simulink model "s_c856m4k_cd"  (R2016b)
(part 21 of 60)

  rx_crc_err_lnk3 : Subsystem  Tag=xps:sw_reg  AncestorBlock=xps_library/software_register  mask(swreg){io_dir=To Processor, io_delay=0, sample_period=1, names=reg, bitwidths=16, bin_pts=0, arith_types=0, sim_port=on, show_format=on}
      mask prompts: io_dir "I/O direction"; io_delay "I/O delay"; sample_period "Sample period"; names "Bitfield names [msb...lsb]"; bitwidths "Bitfield widths"; bin_pts "Bitfield binary pts"; arith_types "Bitfield types, ufix=0, fix=1, bool=2"; sim_port "Provide sim input/output?"; show_format "Print format string?"
      mask help: A 32-bit software-accessible register. Can be divided into bitfields of varying widths and types using the fields in the block mask.
      mask init:
      | swreg_init(gcb)
      settings: AttributesFormatString=1output:uf16.0 = 16 bits
      mask TypeOptions io_dir: To Processor | From Processor
      mask Callback io_dir:
      | mask_enables = get_param(gcb, 'MaskEnables');
      | mask_names = get_param(gcb, 'MaskNames');
      | if strcmp(get_param(gcb, 'io_dir'), 'To Processor'),
      |     mask_enables{ismember(mask_names, 'sample_period')} = 'off';
      | else
      |     mask_enables{ismember(mask_names, 'sample_period')} = 'on';
      | end
      | set_param(gcb, 'MaskEnables', mask_enables);
  second : xbsIndex_r4/Delay  rst=on  infoeditControl=Selection of Reset will increase slice count due to use of real FFs and instead of SRLs  en=on  latency=1  reg_retiming=on  dbl_ovrd=off  block_type=delay
      settings: infoedit=Hardware notes: A delay line is a chain, each link of which is an SRL16 or SRL32 followed by a flip-flop.  block_version=11.4
  sync_delay7 : xbsIndex_r4/Delay  rst=off  infoeditControl=Selection of Reset will increase slice count due to use of real FFs and instead of SRLs  en=off  latency=1  reg_retiming=on  dbl_ovrd=off  block_type=delay
      settings: infoedit=Hardware notes: A delay line is a chain, each link of which is an SRL16 or SRL32 followed by a flip-flop.
  sync_delay9 : xbsIndex_r4/Delay  rst=off  infoeditControl=Selection of Reset will increase slice count due to use of real FFs and instead of SRLs  en=off  latency=1  reg_retiming=on  dbl_ovrd=off  block_type=delay
      settings: infoedit=Hardware notes: A delay line is a chain, each link of which is an SRL16 or SRL32 followed by a flip-flop.
  sync_mon_rst : Subsystem  Tag=xps:sw_reg  AncestorBlock=xps_library/software_register  mask(swreg){io_dir=From Processor, io_delay=0, sample_period=1, names=reg, bitwidths=1, bin_pts=0, arith_types=2, sim_port=on, show_format=on}
      mask prompts: io_dir "I/O direction"; io_delay "I/O delay"; sample_period "Sample period"; names "Bitfield names [msb...lsb]"; bitwidths "Bitfield widths"; bin_pts "Bitfield binary pts"; arith_types "Bitfield types, ufix=0, fix=1, bool=2"; sim_port "Provide sim input/output?"; show_format "Print format string?"
      mask help: A 32-bit software-accessible register. Can be divided into bitfields of varying widths and types using the fields in the block mask.
      mask init:
      | swreg_init(gcb)
      settings: AttributesFormatString=1input:b = 1 bits
      mask TypeOptions io_dir: To Processor | From Processor
      mask Callback io_dir:
      | mask_enables = get_param(gcb, 'MaskEnables');
      | mask_names = get_param(gcb, 'MaskNames');
      | if strcmp(get_param(gcb, 'io_dir'), 'To Processor'),
      |     mask_enables{ismember(mask_names, 'sample_period')} = 'off';
      | else
      |     mask_enables{ismember(mask_names, 'sample_period')} = 'on';
      | end
      | set_param(gcb, 'MaskEnables', mask_enables);
  write_addr_gen_lnk2 : Subsystem
  write_addr_gen_lnk3 : Subsystem
  sync_out : Outport
  q : Outport  Port=2
  dv : Outport  Port=3
  hmc_error : Outport  Port=4
  parity_error : Outport  Port=5
  misco : Outport  Port=6
  tag scope: errstat_lnk2=global, errstat_lnk3=global, hmc_clear_done=global, hmc_clear_win=global, hmc_clear_wraddr_pol0=global, hmc_clear_wraddr_pol1=global, hmc_dout_pol1=global, hmc_dvalid_pol1=global, hmc_init=global, hmc_post=global, hmc_rd_rdy_pol1=global, hmc_tag_out_pol1=global, hmc_wr_rdy_pol1=global, reord_clear_wraddr_pol0=global, rx_crc_err_lnk2=global, rx_crc_err_lnk3=global
  wires:
  Delay37/1 -> Delay36/1
  Delay4/1 -> AddSub/1, Delay1/1
  second/1 -> Delay25/1
  Delay16/1 -> Delay17/1
  Delay21/1 -> Delay16/1
  Delay13/1 -> second/1
  d/1 -> pipeline206/1(d)  "d_in"
  [dout] -> Delay6/1
  pipeline16/1(q) -> hmc/6, Gateway Out103/1  "hmc_tag_in"
  pipeline19/1(q) -> [hmc_dout]  "hmc_dout"
  pipeline20/1(q) -> Convert1/1  "hmc_dvalid"
  pipeline24/1(q) -> [hmc_init]  "init_done"
  pipeline25/1(q) -> [hmc_post]  "post_ok"
  parity_check0/1(dout) -> Gateway Out106/1, pipeline115/1(d)
  addr/1 -> Gateway Out12/1, Delay4/1  "addr"
  pipeline21/1(q) -> [hmc_tag_out]  "hmc_tag_out"
  pipeline22/1(q) -> [hmc_wr_ready]  "wr_ready"
  cd_hmc_rd_tag_err/1(sim_out) -> To Workspace1/1
  addr_stall/1 -> edge_detect9/1(in)  "stall"
  [fifo_dout] -> parity_check0/2(din), Gateway Out21/1
  [fifo_dvalid] -> Gateway Out20/1, parity_check0/1(en)
  parity_check0/2(error) -> pipeline116/1(d)
  sync_delay9/1 -> delay5/1
  delay5/1 -> pipeline114/1(d)
  delay10/1 -> sync_delay7/1
  Constant2/1 -> HMC_reord_bram/5
  Constant3/1 -> HMC_reord_bram/6
  HMC_reord_bram/1 -> Terminator35/1
  Reorder_cntrl/2(bram_rd_en) -> Delay9/1, Gateway Out7/1, HMC_reord_bram/7
  Logical1/1 -> pipeline112/1(d)
  cd_hmc_post/1(sim_out) -> To Workspace10/1
  sync_delay7/1 -> sync_delay9/1
  cd_hmc_post_counter/1(sim_out) -> To Workspace12/1
  Counter2/1 -> cd_hmc_post_counter/1(out_counter)
  cd_hmc_rd_tag_err_count/1(sim_out) -> To Workspace13/1
  cd_hmc_init/1(sim_out) -> To Workspace16/1
  cd_hmc_init_counter/1(sim_out) -> To Workspace17/1
  Counter4/1 -> cd_hmc_init_counter/1(out_counter)
  [hmc_init] -> Inverter2/1
  [hmc_post] -> Inverter6/1
  Inverter2/1 -> Logical1/1
  Inverter6/1 -> Logical1/2
  hmc/11 -> pipeline24/1(d)
  hmc/12 -> pipeline25/1(d)
  hmc/5 -> Gateway Out98/1, pipeline21/1(d)
  hmc/4 -> pipeline23/1(d)
  hmc/3 -> pipeline22/1(d)
  pipeline5/1(q) -> Gateway Out102/1, hmc/5  "hmc_rdadd"
  pipeline17/1(q) -> Gateway Out101/1, hmc/4  "hmc_rin"
  pipeline174/1(q) -> Slice9/1, Slice12/1, hmc/3  "hmc_din"
  pipeline173/1(q) -> hmc/1, Gateway Out100/1  "hmc_win"
  pipeline112/1(q) -> hmc_error/1
  pipeline114/1(q) -> Gateway Out141/1, misco/1
  pipeline115/1(q) -> q/1, Gateway Out85/1, [q_out]
  pipeline116/1(q) -> parity_error/1
  pipeline117/1(q) -> Gateway Out83/1, [q_sync], sync_out/1
  [hmc_post] -> edge_detect2/1, cd_hmc_post/1(out_post)
  [hmc_init] -> edge_detect4/1, cd_hmc_init/1(out_init)
  bus_expand5/1(msb_out8) -> pipeline120/1(d)  "hmc_out1"
  bus_expand5/8(lsb_out1) -> pipeline127/1(d)  "hmc_out8"
  Slice14/1 -> pipeline27/1(d)
  bus_expand8/1(msb_out8) -> pipeline103/1(d)  "hmc_out9"
  bus_expand8/8(lsb_out1) -> pipeline119/1(d)  "hmc_out16"
  Slice15/1 -> pipeline28/1(d)
  pipeline120/1(q) -> hmc_reord0/1(in_d00)
  pipeline121/1(q) -> hmc_reord0/2(in_d01)
  pipeline122/1(q) -> hmc_reord0/3(in_d02)
  pipeline124/1(q) -> hmc_reord0/5(in_d04)
  pipeline125/1(q) -> hmc_reord0/6(in_d05)
  pipeline126/1(q) -> hmc_reord0/7(in_d06)
  pipeline128/1(q) -> hmc_reord0/11(we)
  pipeline137/1(q) -> hmc_reord0/12(trig)
  pipeline119/1(q) -> hmc_reord1/8(in_d07)
  pipeline118/1(q) -> hmc_reord1/7(in_d06)
  pipeline111/1(q) -> hmc_reord1/6(in_d05)
  pipeline107/1(q) -> hmc_reord1/5(in_d04)
  pipeline106/1(q) -> hmc_reord1/4(in_d03)
  pipeline105/1(q) -> hmc_reord1/3(in_d02)
  pipeline104/1(q) -> hmc_reord1/2(in_d01)
  pipeline103/1(q) -> hmc_reord1/1(in_d00)
  bus_expand5/2(out7) -> pipeline121/1(d)
  bus_expand5/4(out5) -> pipeline123/1(d)
  bus_expand5/7(out2) -> pipeline126/1(d)
  bus_expand5/3(out6) -> pipeline122/1(d)
  bus_expand8/7(out2) -> pipeline118/1(d)
  bus_expand5/5(out4) -> pipeline124/1(d)
  bus_expand5/6(out3) -> pipeline125/1(d)
  bus_expand8/5(out4) -> pipeline107/1(d)
  bus_expand8/4(out5) -> pipeline106/1(d)
  bus_expand8/6(out3) -> pipeline111/1(d)
  bus_expand8/3(out6) -> pipeline105/1(d)
  bus_expand8/2(out7) -> pipeline104/1(d)
  [hmc_reord_data] -> Slice15/1, Slice14/1
  pipeline127/1(q) -> hmc_reord0/8(in_d07)
  pipeline123/1(q) -> hmc_reord0/4(in_d03)
  Constant12/1 -> Relational5/2
  [hmc_win_pol0] -> Counter7/2
  Register4/1 -> pipeline156/1(d)
  data_in_counter/1(sim_out) -> To Workspace25/1
  [hmc_dvalid] -> Counter9/2
  Register10/1 -> pipeline155/1(d)
  data_out_counter/1(sim_out) -> To Workspace26/1
  Relational5/1 -> Delay3/1, Register10/2, Register4/2, Delay5/1
  Counter9/1 -> Register10/1
  Counter7/1 -> Register4/1
  pipeline155/1(q) -> data_out_counter/1(out_counter)
  pipeline156/1(q) -> data_in_counter/1(out_counter)
  Counter6/1 -> Relational5/1
  pipeline159/1(q) -> Gateway Out3/1, [radd]
  pipeline162/1(q) -> Gateway Out91/1, [din]
  Delay17/1 -> Delay24/1
  pipeline167/1(q) -> Gateway Out46/1, hmc/7
  pipeline168/1(q) -> Gateway Out47/1, hmc/8
  pipeline169/1(q) -> Gateway Out49/1, hmc/9
  pipeline170/1(q) -> Gateway Out51/1, hmc/10
  pipeline171/1(q) -> Gateway Out52/1, hmc/11
  pipeline172/1(q) -> Gateway Out53/1, hmc/12
  bus_expand13/2(out7) -> Gateway Out73/1
  bus_expand13/3(out6) -> Gateway Out74/1
  bus_expand13/4(out5) -> Gateway Out75/1
  bus_expand13/5(out4) -> Gateway Out76/1
  bus_expand13/6(out3) -> Gateway Out77/1
  bus_expand13/7(out2) -> Gateway Out78/1
  bus_expand13/8(lsb_out1) -> Gateway Out79/1
  Gateway Out79/1 -> To Workspace74/1
  Gateway Out78/1 -> To Workspace73/1
  Gateway Out77/1 -> To Workspace72/1
  Gateway Out76/1 -> To Workspace71/1
  Gateway Out75/1 -> To Workspace70/1
  Gateway Out74/1 -> To Workspace69/1
  Gateway Out73/1 -> To Workspace67/1
  [q_out] -> bus_expand13/1(bus_in)
  bus_expand13/1(msb_out8) -> Gateway Out80/1
  Gateway Out80/1 -> To Workspace68/1
  bus_expand2/1(msb_out8) -> pipeline26/1(d)  "hmc_out9"
  bus_expand2/8(lsb_out1) -> pipeline36/1(d)  "hmc_out16"
  [fifo_dout] -> Slice3/1
  pipeline36/1(q) -> fifo0/8(in_d07)
  pipeline35/1(q) -> fifo0/7(in_d06)
  pipeline34/1(q) -> fifo0/6(in_d05)
  pipeline33/1(q) -> fifo0/5(in_d04)
  pipeline32/1(q) -> fifo0/4(in_d03)
  pipeline31/1(q) -> fifo0/3(in_d02)
  pipeline30/1(q) -> fifo0/2(in_d01)
  pipeline26/1(q) -> fifo0/1(in_d00)
  bus_expand2/7(out2) -> pipeline35/1(d)
  bus_expand2/5(out4) -> pipeline33/1(d)
  bus_expand2/4(out5) -> pipeline32/1(d)
  bus_expand2/6(out3) -> pipeline34/1(d)
  bus_expand2/3(out6) -> pipeline31/1(d)
  bus_expand2/2(out7) -> pipeline30/1(d)
  pipeline56/1(q) -> fifo0/13(trig)
  pipeline57/1(q) -> fifo0/12(we)
  [mux_sel] -> pipeline55/1(d)
  pipeline72/1(q) -> fifo0/9(in_mux_sel)
  hmc_delay/1(sim_out) -> To Workspace5/1
  [hmc_delay] -> Convert4/1
  Convert4/1 -> hmc_delay/1(out_delay)
  [sys_rst] -> Reorder_cntrl/1(rst)
  Gateway Out22/1 -> To Workspace9/1
  Slice8/1 -> bus_expand4/1(bus_in)
  [hmc_reord_data] -> Slice8/1
  bus_expand4/1(msb_out8) -> Gateway Out22/1
  Gateway Out24/1 -> To Workspace11/1
  Gateway Out25/1 -> To Workspace18/1
  Gateway Out26/1 -> To Workspace19/1
  bus_expand4/4(out5) -> Gateway Out26/1
  bus_expand4/3(out6) -> Gateway Out25/1
  bus_expand4/2(out7) -> Gateway Out24/1
  Gateway Out27/1 -> To Workspace21/1
  bus_expand4/5(out4) -> Gateway Out27/1
  Gateway Out28/1 -> To Workspace22/1
  bus_expand4/6(out3) -> Gateway Out28/1
  Gateway Out29/1 -> To Workspace23/1
  bus_expand4/7(out2) -> Gateway Out29/1
  Gateway Out30/1 -> To Workspace24/1
  bus_expand4/8(lsb_out1) -> Gateway Out30/1
  Slice10/1 -> bus_expand6/1(bus_in)
  [hmc_reord_data] -> Slice10/1
  Gateway Out31/1 -> To Workspace77/1
  Gateway Out32/1 -> To Workspace27/1
  Gateway Out33/1 -> To Workspace28/1
  Gateway Out35/1 -> To Workspace29/1
  Gateway Out37/1 -> To Workspace31/1
  Gateway Out38/1 -> To Workspace32/1
  Gateway Out39/1 -> To Workspace33/1
  Gateway Out42/1 -> To Workspace36/1
  bus_expand6/1(msb_out8) -> Gateway Out31/1
  bus_expand6/2(out7) -> Gateway Out32/1
  bus_expand6/3(out6) -> Gateway Out33/1
  bus_expand6/4(out5) -> Gateway Out35/1
  bus_expand6/5(out4) -> Gateway Out37/1
  bus_expand6/6(out3) -> Gateway Out38/1
  bus_expand6/7(out2) -> Gateway Out39/1
  bus_expand6/8(lsb_out1) -> Gateway Out42/1
  Gateway Out99/1 -> To Workspace94/1
  Gateway Out100/1 -> To Workspace95/1
  Gateway Out101/1 -> To Workspace96/1
  Gateway Out102/1 -> To Workspace97/1
  Gateway Out103/1 -> To Workspace98/1
  cd_hmc_sync_in/1(sim_out) -> To Workspace102/1
  cd_hmc_sync_out/1(sim_out) -> To Workspace101/1
  pipeline81/1(q) -> Register1/3, Register1/1
  pipeline82/1(q) -> Register5/3, Register5/1
  Register5/1 -> pipeline132/1(d)
  pipeline102/1(q) -> Register1/2
  pipeline108/1(q) -> Register5/2
  cd_hmc_sync_in_cnt/1(sim_out) -> To Workspace104/1
  Counter10/1 -> pipeline129/1(d)
  cd_hmc_sync_out_cnt/1(sim_out) -> To Workspace105/1
  Counter11/1 -> pipeline113/1(d)
  pipeline113/1(q) -> cd_hmc_sync_out_cnt/1(out_reg)
  pipeline129/1(q) -> cd_hmc_sync_in_cnt/1(out_reg)
  pipeline131/1(q) -> cd_hmc_sync_in/1(out_reg)
  pipeline132/1(q) -> cd_hmc_sync_out/1(out_reg)
  pipeline146/1(q) -> cd_hmc_rd_tag_err_count/1(out_counter)
  pipeline165/1(q) -> cd_hmc_rd_tag_err/1(out_error)
  Register1/1 -> pipeline131/1(d)
  sync_mon_rst/1(in_reg) -> pipeline98/1(d)
  Constant18/1 -> sync_mon_rst/1(sim_1)
  pipeline91/1(q) -> Counter11/1
  pipeline110/1(q) -> Counter11/2
  pipeline90/1(q) -> Counter10/1
  pipeline109/1(q) -> Counter10/2
  Gateway Out19/1 -> To Workspace4/1
  pipeline3/1(q) -> hmc/2, Gateway Out99/1  "hmc_wadd"
  hmc/1 -> Slice42/1, Slice43/1, pipeline19/1(d), Slice6/1, Slice13/1
  Slice13/1 -> Convert16/1
  Gateway Out87/1 -> To Workspace82/1
  [hmc_win_p0] -> pipeline173/1(d)
  Gateway Out90/1 -> To Workspace85/1
  read_tag_check/1(rd_tag_err) -> pipeline165/1(d)
  read_tag_check/2(rd_tag_err_count) -> pipeline146/1(d)
  cd_hmc_wr_req_count/1(sim_out) -> To Workspace115/1
  Counter3/1 -> pipeline4/1(d)
  pipeline4/1(q) -> cd_hmc_wr_req_count/1(out_reg)
  pipeline18/1(q) -> Counter3/1
  pipeline166/1(q) -> Counter3/2
  cd_hmc_rd_req_count/1(sim_out) -> To Workspace116/1
  Counter12/1 -> pipeline177/1(d)
  pipeline177/1(q) -> cd_hmc_rd_req_count/1(out_reg)
  pipeline176/1(q) -> Counter12/1
  pipeline175/1(q) -> Counter12/2
  [hmc_dvalid] -> pipeline183/1(d)  "tp2"
  [hmc_tag_out] -> pipeline180/1(d)  "tp1"
  [hmc_tag_pol0] -> pipeline181/1(d)
  [hmc_sync] -> pipeline182/1(d)
  pipeline181/1(q) -> read_tag_check/1(HMC_tag_in)
  pipeline180/1(q) -> read_tag_check/2(HMC_tag_out)
  pipeline183/1(q) -> read_tag_check/3(HMC_dvalid)
  pipeline182/1(q) -> read_tag_check/4(HMC_sync)
  cd_hmc_rd_dvalid_count/1(sim_out) -> To Workspace119/1
  Counter13/1 -> pipeline186/1(d)
  pipeline186/1(q) -> cd_hmc_rd_dvalid_count/1(out_reg)
  pipeline185/1(q) -> Counter13/1
  pipeline184/1(q) -> Counter13/2
  Constant20/1 -> dvalid_capture_cntrl/1(sim_1)
  dvalid_capture_cntrl/1(in_reg) -> pipeline78/1(d)
  Logical15/1 -> edge_detect28/1
  [hmc_dvalid] -> pipeline220/1(d)
  Logical/1 -> edge_detect24/1
  [hmc_rin_pol0] -> pipeline217/1(d)
  Logical16/1 -> edge_detect33/1
  [hmc_win_pol0] -> pipeline214/1(d)
  pipeline76/1(q) -> Logical16/1
  pipeline77/1(q) -> Logical/1
  pipeline75/1(q) -> Logical15/1
  pipeline78/1(q) -> [capture_cntrl]
  [capture_cntrl] -> pipeline75/1(d)
  [capture_cntrl] -> pipeline77/1(d)
  [capture_cntrl] -> pipeline76/1(d)
  pipeline83/1(q) -> read_tag_check/5(Capture_cntrl)
  [capture_cntrl] -> pipeline83/1(d)
  pipeline213/1(q) -> pipeline18/1(d)
  pipeline219/1(q) -> pipeline185/1(d)
  pipeline216/1(q) -> pipeline176/1(d)
  Constant22/1 -> dvalid_capture_cntrl_rst/1(sim_1)
  dvalid_capture_cntrl_rst/1(in_reg) -> pipeline84/1(d)
  pipeline84/1(q) -> edge_detect16/1
  [sync_mon_rst] -> pipeline216/1(d)
  [sync_mon_rst] -> pipeline219/1(d)
  [sync_mon_rst] -> pipeline213/1(d)
  cd_reord_sync_out/1(sim_out) -> To Workspace117/1
  Register12/1 -> pipeline85/1(d)
  [sync_mon_rst] -> edge_detect1/1
  pipeline85/1(q) -> cd_reord_sync_out/1(out_reg)
  pipeline86/1(q) -> Register12/3, Register12/1
  [sync_mon_rst] -> edge_detect31/1
  pipeline98/1(q) -> edge_detect11/1
  cd_reord_sync_cnt/1(sim_out) -> To Workspace118/1
  Counter14/1 -> pipeline88/1(d)
  pipeline88/1(q) -> cd_reord_sync_cnt/1(out_reg)
  pipeline87/1(q) -> Counter14/2
  pipeline92/1(q) -> Register12/2
  pipeline89/1(q) -> Counter14/1
  [hmc_rin_p0] -> pipeline17/1(d)
  [hmc_tag_p0] -> pipeline16/1(d)
  cd_hmc_sync/1(sim_out) -> To Workspace112/1
  Counter15/1 -> pipeline95/1(d)
  pipeline95/1(q) -> cd_hmc_sync/1(out_reg)
  pipeline94/1(q) -> Counter15/1
  pipeline93/1(q) -> Counter15/2
  [hmc_sync] -> pipeline211/1(d)
  [sync_mon_rst] -> pipeline210/1(d)
  pipeline210/1(q) -> edge_detect23/1
  pipeline211/1(q) -> edge_detect17/1
  Gateway Out98/1 -> To Workspace100/1
  Gateway Out105/1 -> To Workspace109/1
  hmc/2 -> Gateway Out105/1, Logical34/2, pipeline20/1(d)
  [wadd] -> hmc_control/1(waddr)
  [hmc_delay] -> hmc_control/2(delay)
  [hmc_sync] -> hmc_control/3(sync_in)
  [win] -> hmc_control/4(win)
  [rin] -> hmc_control/5(rin)
  [radd] -> hmc_control/6(rdadd)
  [din] -> hmc_control/7(din)
  hmc_control/3(hmc_rin) -> [hmc_rin_pol0]
  hmc_control/4(hmc_raddr) -> [hmc_raddr_pol0]
  hmc_control/6(hmc_tag) -> [hmc_tag_pol0]
  [hmc_rin_pol0] -> pipeline198/1(d)
  [hmc_tag_out] -> pipeline193/1(d)
  [hmc_tag_pol0] -> pipeline196/1(d)
  [hmc_raddr_pol0] -> pipeline197/1(d)
  [hmc_rd_rdy] -> pipeline194/1(d)
  [hmc_dvalid] -> pipeline195/1(d)
  pipeline193/1(q) -> pipeline100/1(d)
  pipeline194/1(q) -> pipeline99/1(d)
  pipeline195/1(q) -> pipeline96/1(d)
  pipeline196/1(q) -> pipeline8/1(d)
  pipeline197/1(q) -> pipeline7/1(d)
  pipeline198/1(q) -> pipeline6/1(d)
  pipeline199/1(q) -> [rin], Gateway Out4/1
  [hmc_wr_ready] -> pipeline200/1(d)
  pipeline200/1(q) -> pipeline201/1(d)
  [hmc_win_pol0] -> pipeline203/1(d)
  [hmc_waddr_pol0] -> pipeline202/1(d)
  pipeline202/1(q) -> pipeline204/1(d)
  pipeline203/1(q) -> pipeline205/1(d)
  Delay28/1 -> Delay31/1
  Gateway Out1/1 -> To Workspace6/1
  Gateway Out2/1 -> To Workspace7/1
  Gateway Out3/1 -> To Workspace8/1
  Gateway Out4/1 -> To Workspace20/1
  pipeline214/1(q) -> Logical16/2
  pipeline217/1(q) -> Logical/2
  pipeline220/1(q) -> Logical15/2
  pipeline9/1(q) -> Logical27/1
  Logical31/1 -> pipeline50/1(d)
  pipeline2/1(q) -> [hmc_delay]
  pipeline206/1(q) -> [dout]
  pipeline12/1(q) -> Delay23/1
  Logical32/1 -> edge_detect13/1(in)
  Logical29/1 -> edge_detect5/1(in)
  Delay36/1 -> Delay33/1
  pipeline23/1(q) -> [hmc_rd_rdy]  "rd_ready"
  AddSub/1 -> Delay32/1  "rd_add_HR"
  Gateway Out6/1 -> To Workspace75/1
  Reorder_cntrl/1(bram_rd_addr) -> Gateway Out6/1, HMC_reord_bram/4
  Gateway Out7/1 -> To Workspace76/1
  [reord_addr] -> Reorder_cntrl/2(tag)
  Gateway Out13/1 -> To Workspace84/1
  Gateway Out11/1 -> To Workspace81/1
  pipeline209/1(q) -> [hmc_sync], Gateway Out19/1
  [reord_wea] -> Gateway Out13/1, Logical10/1, HMC_reord_bram/3
  Convert1/1 -> [hmc_dvalid]
  pipeline1/1(q) -> Delay37/1
  pipeline79/1(q) -> [q_dvalid], Gateway Out84/1, dv/1
  hmc_wr_err/1(sim_out) -> To Workspace136/1
  Counter16/1 -> pipeline10/1(d)
  pipeline10/1(q) -> hmc_wr_err/1(out_reg)
  pipeline223/1(q) -> Counter16/1
  [sync_mon_rst] -> edge_detect26/1
  [hmc_wr_ready] -> Inverter/1
  Inverter/1 -> Logical5/1
  pipeline224/1(q) -> Counter16/2
  Logical5/1 -> pipeline224/1(d)
  hmc_rd_err/1(sim_out) -> To Workspace137/1
  Counter17/1 -> pipeline225/1(d)
  pipeline225/1(q) -> hmc_rd_err/1(out_reg)
  pipeline226/1(q) -> Counter17/1
  [sync_mon_rst] -> edge_detect15/1
  [hmc_rd_rdy] -> Inverter12/1
  Inverter12/1 -> Logical6/1
  pipeline227/1(q) -> Counter17/2
  Logical6/1 -> pipeline227/1(d)
  Delay33/1 -> pipeline209/1(d)
  Delay32/1 -> pipeline159/1(d)
  Delay31/1 -> Logical13/1, pipeline232/1(d), pipeline199/1(d)
  Delay25/1 -> pipeline162/1(d)
  Gateway Out20/1 -> To Workspace91/1
  Gateway Out21/1 -> To Workspace92/1
  [hmc_reord_sync] -> pipeline86/1(d), pipeline87/1(d)
  Slice24/1 -> Convert23/1
  Convert24/1 -> Logical33/2
  Convert23/1 -> Logical33/1
  Slice25/1 -> Convert24/1
  Logical33/1 -> Convert25/1
  Convert25/1 -> edge_detect32/1
  [fifo_sync] -> delay1/1  "sync"
  Gateway Out82/1 -> To Workspace108/1
  HMC_reord_bram/2 -> Delay2/1, Slice25/1, Slice24/1
  Gateway Out23/1 -> To Workspace93/1
  Gateway Out83/1 -> To Workspace110/1
  Gateway Out84/1 -> To Workspace111/1
  Gateway Out85/1 -> To Workspace113/1
  [fifo_dvalid] -> delay8/1
  Logical27/1 -> addr_stall/2
  misci/1 -> Gateway Out138/1, Delay21/1, Slice29/1
  [sync_in] -> pipeline1/1(d)
  en/1 -> Gateway Out140/1, [en_in]  "en_in"
  Delay70/1 -> pipeline233/1(d)
  AddSub2/1 -> Gateway Out181/1, AddSub/2
  Constant/1 -> AddSub2/2
  [delay_in] -> AddSub2/1
  Slice29/1 -> [ld_val]
  pipeline232/1(q) -> Gateway Out2/1, [win]
  delay/1 -> Register13/1, Gateway Out176/1  "delay"
  Register13/1 -> Gateway Out166/1, [delay_in], pipeline2/1(d)
  hmc_wr_rd_rdy_clash/1(sim_out) -> To Workspace124/1
  Counter20/1 -> pipeline207/1(d)
  pipeline207/1(q) -> hmc_wr_rd_rdy_clash/1(out_reg)
  pipeline208/1(q) -> Counter20/1
  pipeline231/1(q) -> Counter20/2
  [sync_mon_rst] -> edge_detect14/1
  [hmc_rd_rdy] -> Logical19/2
  [hmc_wr_ready] -> Logical19/1
  Logical19/1 -> pipeline231/1(d)
  Gateway Out91/1 -> To Workspace125/1
  Gateway Out93/1 -> To Workspace126/1
  Gateway Out106/1 -> To Workspace132/1
  Gateway Out107/1 -> To Workspace133/1
  Gateway Out108/1 -> To Workspace134/1
  pipeline233/1(q) -> Gateway Out1/1, [wadd]
  Delay1/1 -> Delay70/1
  delay1/1 -> pipeline117/1(d), Gateway Out108/1
  delay8/1 -> pipeline79/1(d), Gateway Out107/1
  Delay2/1 -> Gateway Out93/1, [hmc_reord_data]
  delay4/1 -> Gateway Out23/1, [fifo_sync]
  [sync_mon_rst] -> edge_detect18/1
  edge_detect31/1 -> pipeline102/1(d), pipeline90/1(d)
  edge_detect12/1 -> pipeline109/1(d), pipeline81/1(d)
  edge_detect18/1 -> pipeline45/1(d), pipeline108/1(d), pipeline91/1(d)
  edge_detect20/1 -> pipeline82/1(d), pipeline110/1(d)
  edge_detect32/1 -> Delay8/1
  edge_detect1/1 -> pipeline89/1(d), pipeline92/1(d)
  edge_detect15/1 -> pipeline226/1(d)
  edge_detect26/1 -> pipeline223/1(d)
  edge_detect14/1 -> pipeline208/1(d)
  edge_detect16/1 -> [capture_cntrl_rst]
  edge_detect13/1(out) -> Gateway Out8/1, pipeline160/1(d), pipeline161/1(d), pipeline157/1(d)
  edge_detect23/1 -> pipeline94/1(d)
  edge_detect17/1 -> pipeline93/1(d)
  edge_detect2/1 -> Counter2/1
  edge_detect4/1 -> Counter4/1
  Delay3/1 -> Counter9/1
  Delay5/1 -> Counter7/1
  Slice6/1 -> Convert30/1
  Convert30/1 -> Logical20/1
  Convert16/1 -> Logical20/2
  Slice9/1 -> Convert11/1
  Slice12/1 -> Convert31/1
  Convert31/1 -> Gateway Out178/1, Logical28/1
  Convert11/1 -> Gateway Out177/1, Logical28/2
  Logical28/1 -> edge_detect12/1, Gateway Out90/1
  Slice27/1 -> Convert32/1
  Slice16/1 -> Convert33/1
  Convert33/1 -> Logical29/1
  Convert32/1 -> Logical29/2
  [hmc_dout] -> Slice27/1, Slice16/1
  Slice2/1 -> Convert5/1
  Slice1/1 -> Convert6/1
  Convert6/1 -> Gateway Out9/1, Logical32/1
  Convert5/1 -> Gateway Out14/1, Logical32/2
  [hmc_din_pol0] -> Slice2/1, Slice1/1
  Delay6/1 -> Delay13/1
  Delay8/1 -> Gateway Out82/1, [hmc_reord_sync]
  [hmc_win_p1] -> pipeline167/1(d)
  [hmc_waddr_p1] -> pipeline168/1(d)
  [hmc_din_p1] -> pipeline169/1(d)
  [hmc_rin_p1] -> pipeline170/1(d)
  [hmc_raddr_p1] -> pipeline171/1(d)
  [hmc_tag_p1] -> pipeline172/1(d)
  hmc/7 -> Gateway Out56/1, pipeline61/1(d)
  hmc/6 -> Gateway Out55/1, pipeline11/1(d)
  hmc/8 -> pipeline152/1(d)
  hmc/9 -> pipeline153/1(d)
  hmc/10 -> Gateway Out54/1, pipeline154/1(d)
  pipeline154/1(q) -> [hmc_tag_out_pol1]
  pipeline153/1(q) -> [hmc_rd_rdy_pol1]
  pipeline152/1(q) -> [hmc_wr_rdy_pol1]
  pipeline61/1(q) -> [hmc_dvalid_pol1]
  pipeline11/1(q) -> [hmc_dout_pol1]
  [hmc_din_p0] -> pipeline174/1(d)
  Register14/1 -> pipeline260/1(d), pipeline271/1(d), pipeline178/1(d)
  [hmc_win_pol0] -> Register14/3, Register14/1
  [sync_mon_rst] -> edge_detect19/1(in)
  [hmc_dvalid] -> Register15/3, Register15/1
  [sync_mon_rst] -> edge_detect21/1(in)
  edge_detect19/1(out) -> Register14/2
  edge_detect21/1(out) -> Register15/2
  Gateway Out46/1 -> To Workspace39/1
  Gateway Out47/1 -> To Workspace40/1
  Gateway Out49/1 -> To Workspace42/1
  Gateway Out51/1 -> To Workspace44/1
  Gateway Out52/1 -> To Workspace45/1
  Gateway Out53/1 -> To Workspace46/1
  Gateway Out54/1 -> To Workspace47/1
  Gateway Out55/1 -> To Workspace48/1
  Gateway Out56/1 -> To Workspace49/1
  bus_expand3/1(msb_out8) -> pipeline252/1(d)  "hmc_out1"
  bus_expand3/8(lsb_out1) -> pipeline259/1(d)  "hmc_out8"
  Slice28/1 -> bus_expand3/1(bus_in)
  bus_expand7/1(msb_out8) -> pipeline244/1(d)  "hmc_out9"
  bus_expand7/8(lsb_out1) -> pipeline251/1(d)  "hmc_out16"
  Slice30/1 -> bus_expand7/1(bus_in)
  pipeline252/1(q) -> hmc_din0_p0/1(in_d00)
  pipeline253/1(q) -> hmc_din0_p0/2(in_d01)
  pipeline254/1(q) -> hmc_din0_p0/3(in_d02)
  pipeline256/1(q) -> hmc_din0_p0/5(in_d04)
  pipeline257/1(q) -> hmc_din0_p0/6(in_d05)
  pipeline258/1(q) -> hmc_din0_p0/7(in_d06)
  pipeline260/1(q) -> hmc_din0_p0/9(we)
  pipeline160/1(q) -> hmc_din0_p0/10(trig)
  pipeline251/1(q) -> hmc_din1_p0/8(in_d07)
  pipeline250/1(q) -> hmc_din1_p0/7(in_d06)
  pipeline249/1(q) -> hmc_din1_p0/6(in_d05)
  pipeline248/1(q) -> hmc_din1_p0/5(in_d04)
  pipeline247/1(q) -> hmc_din1_p0/4(in_d03)
  pipeline246/1(q) -> hmc_din1_p0/3(in_d02)
  pipeline245/1(q) -> hmc_din1_p0/2(in_d01)
  pipeline244/1(q) -> hmc_din1_p0/1(in_d00)
  bus_expand3/2(out7) -> pipeline253/1(d)
  bus_expand3/4(out5) -> pipeline255/1(d)
  bus_expand3/7(out2) -> pipeline258/1(d)
  bus_expand3/3(out6) -> pipeline254/1(d)
  bus_expand7/7(out2) -> pipeline250/1(d)
  bus_expand3/5(out4) -> pipeline256/1(d)
  bus_expand3/6(out3) -> pipeline257/1(d)
  bus_expand7/5(out4) -> pipeline248/1(d)
  bus_expand7/4(out5) -> pipeline247/1(d)
  bus_expand7/6(out3) -> pipeline249/1(d)
  bus_expand7/3(out6) -> pipeline246/1(d)
  bus_expand7/2(out7) -> pipeline245/1(d)
  [hmc_din_pol0] -> pipeline212/1(d), pipeline164/1(d)
  pipeline164/1(q) -> Slice30/1
  pipeline259/1(q) -> hmc_din0_p0/8(in_d07)
  pipeline255/1(q) -> hmc_din0_p0/4(in_d03)
  pipeline271/1(q) -> hmc_din1_p0/9(we)
  pipeline161/1(q) -> hmc_din1_p0/10(trig)
  pipeline212/1(q) -> Slice28/1
  edge_detect5/1(out) -> pipeline215/1(d), pipeline42/1(d), pipeline221/1(d)
  Register15/1 -> pipeline41/1(d), pipeline266/1(d), pipeline265/1(d)
  bus_expand9/1(msb_out8) -> pipeline240/1(d)  "hmc_out1"
  bus_expand9/8(lsb_out1) -> pipeline264/1(d)  "hmc_out8"
  Slice4/1 -> bus_expand9/1(bus_in)
  bus_expand10/1(msb_out8) -> pipeline229/1(d)  "hmc_out9"
  bus_expand10/8(lsb_out1) -> pipeline239/1(d)  "hmc_out16"
  Slice26/1 -> bus_expand10/1(bus_in)
  pipeline240/1(q) -> hmc_dout0_p0/1(in_d00)
  pipeline241/1(q) -> hmc_dout0_p0/2(in_d01)
  pipeline242/1(q) -> hmc_dout0_p0/3(in_d02)
  pipeline261/1(q) -> hmc_dout0_p0/5(in_d04)
  pipeline262/1(q) -> hmc_dout0_p0/6(in_d05)
  pipeline263/1(q) -> hmc_dout0_p0/7(in_d06)
  pipeline265/1(q) -> hmc_dout0_p0/9(we)
  pipeline215/1(q) -> hmc_dout0_p0/10(trig)
  pipeline239/1(q) -> hmc_dout1_p0/8(in_d07)
  pipeline238/1(q) -> hmc_dout1_p0/7(in_d06)
  pipeline237/1(q) -> hmc_dout1_p0/6(in_d05)
  pipeline236/1(q) -> hmc_dout1_p0/5(in_d04)
  pipeline235/1(q) -> hmc_dout1_p0/4(in_d03)
  pipeline234/1(q) -> hmc_dout1_p0/3(in_d02)
  pipeline230/1(q) -> hmc_dout1_p0/2(in_d01)
  pipeline229/1(q) -> hmc_dout1_p0/1(in_d00)
  bus_expand9/2(out7) -> pipeline241/1(d)
  bus_expand9/4(out5) -> pipeline243/1(d)
  bus_expand9/7(out2) -> pipeline263/1(d)
  bus_expand9/3(out6) -> pipeline242/1(d)
  bus_expand10/7(out2) -> pipeline238/1(d)
  bus_expand9/5(out4) -> pipeline261/1(d)
  bus_expand9/6(out3) -> pipeline262/1(d)
  bus_expand10/5(out4) -> pipeline236/1(d)
  bus_expand10/4(out5) -> pipeline235/1(d)
  bus_expand10/6(out3) -> pipeline237/1(d)
  bus_expand10/3(out6) -> pipeline234/1(d)
  bus_expand10/2(out7) -> pipeline230/1(d)
  [hmc_dout] -> pipeline222/1(d), pipeline228/1(d)
  pipeline222/1(q) -> Slice26/1
  pipeline264/1(q) -> hmc_dout0_p0/8(in_d07)
  pipeline243/1(q) -> hmc_dout0_p0/4(in_d03)
  pipeline266/1(q) -> hmc_dout1_p0/9(we)
  pipeline221/1(q) -> hmc_dout1_p0/10(trig)
  pipeline228/1(q) -> Slice4/1
  Convert2/1 -> Gateway Out10/1, Delay28/1, addr/2
  addr_stall1/1 -> Slice31/1  "stall"
  Convert3/1 -> addr1/2, Gateway Out5/1, [hmc_clear_win]
  [hmc_init] -> Logical7/1
  [hmc_post] -> Logical7/2
  Logical7/1 -> Logical11/2, Delay11/1, reord_clear/2
  Delay11/1 -> addr_stall1/2
  [clear_hmc_addr_range] -> Relational/2
  Relational/1 -> Gateway Out16/1, Register/3, Register/1
  [hmc_clear_done] -> Gateway Out96/1, Mux1/1
  [hmc_clear_done] -> Mux2/1
  [hmc_clear_wraddr_pol0] -> Mux1/2
  Mux1/1 -> Gateway Out109/1, [hmc_waddr_p0]
  hmc_control/1(hmc_wraddr) -> [hmc_waddr_pol0]
  Mux2/1 -> Gateway Out110/1, [hmc_win_p0]
  hmc_control/2(hmc_win) -> [hmc_win_pol0]
  [hmc_clear_done] -> Mux3/1
  Mux3/1 -> Gateway Out111/1, [hmc_din_p0]
  hmc_control/5(hmc_din_256) -> [hmc_din_pol0]
  Constant4/1 -> Mux3/2
  [hmc_clear_win] -> Mux2/2
  Gateway Out96/1 -> To Workspace128/1
  Gateway Out109/1 -> To Workspace131/1
  Gateway Out110/1 -> To Workspace135/1
  Gateway Out111/1 -> To Workspace138/1
  [hmc_clear_done] -> Mux4/1
  [hmc_clear_done] -> Mux5/1
  [hmc_clear_wraddr_pol1] -> Mux4/2
  [hmc_waddr_pol1] -> Mux4/3
  Mux4/1 -> [hmc_waddr_p1], Gateway Out112/1
  Mux5/1 -> [hmc_win_p1], Gateway Out113/1
  [hmc_win_pol1] -> Mux5/3
  [hmc_clear_done] -> Mux6/1
  Mux6/1 -> [hmc_din_p1], Gateway Out114/1
  [hmc_din_pol1] -> Mux6/3
  Constant5/1 -> Mux6/2
  [hmc_clear_win] -> Mux5/2
  Gateway Out112/1 -> To Workspace140/1
  Gateway Out113/1 -> To Workspace141/1
  Gateway Out114/1 -> To Workspace142/1
  [hmc_waddr_pol0] -> Mux1/3
  [hmc_win_pol0] -> Mux2/3
  [hmc_din_pol0] -> Mux3/3
  Logical11/1 -> edge_detect22/1
  clear_hmc/1(in_reg) -> pipeline267/1(d)
  [clear_hmc] -> Logical11/1
  pipeline267/1(q) -> edge_detect25/1
  Gateway Out116/1 -> To Workspace143/1
  Constant8/1 -> clear_hmc/1(sim_1)
  edge_detect25/1 -> [clear_hmc]
  Slice31/1 -> edge_detect27/1
  Gateway Out117/1 -> To Workspace144/1
  [hmc_clear_done] -> pipeline268/1(d)
  pipeline268/1(q) -> hmc_clear_done/1(out_level)
  hmc_clear_done/1(sim_out) -> To Workspace145/1
  edge_detect27/1 -> Convert3/1, Gateway Out117/1
  Logical20/1 -> Gateway Out118/1, Logical34/1, edge_detect8/1
  Logical34/1 -> edge_detect20/1, Gateway Out87/1
  Gateway Out118/1 -> To Workspace146/1
  Slice32/1 -> Convert18/1
  Convert26/1 -> Logical36/2
  Convert18/1 -> Logical36/1
  Slice33/1 -> Convert26/1
  Logical36/1 -> Logical10/2, Convert27/1
  Convert27/1 -> edge_detect3/1
  Gateway Out119/1 -> To Workspace147/1
  edge_detect3/1 -> Gateway Out119/1
  [hmc_reord_sync] -> pipeline140/1(d)
  pipeline138/1(q) -> hmc_reord1/11(we)
  pipeline144/1(q) -> hmc_reord1/12(trig)
  [hmc_reord_dvalid] -> Register16/1, Register16/3, pipeline139/1(d)
  [sync_mon_rst] -> edge_detect6/1(in)
  edge_detect6/1(out) -> Register16/2, Register17/2
  Register16/1 -> Convert37/1
  [hmc_reord_dvalid] -> pipeline29/1(d), Register17/3, Register17/1
  [hmc_reord_sync] -> pipeline80/1(d)
  Register17/1 -> Convert36/1
  Convert36/1 -> pipeline138/1(d)
  Convert37/1 -> pipeline128/1(d)
  sync/1 -> Gateway Out139/1, [sync_in]  "sync_in"
  pipeline54/1(q) -> hmc_reord0/10(in_sync)
  pipeline48/1(q) -> hmc_reord0/9(in_dvalid)
  pipeline150/1(q) -> hmc_reord1/10(in_sync)
  pipeline149/1(q) -> hmc_reord1/9(in_dvalid)
  pipeline269/1(q) -> fifo0/10(in_dvalid)
  pipeline270/1(q) -> fifo0/11(in_sync)
  [hmc_win_p0] -> Logical5/2
  [hmc_rin_p0] -> Logical6/2
  Gateway Out48/1 -> To Workspace164/1
  Slice35/1 -> bus_expand14/1(bus_in)
  [hmc_din_p0] -> pipeline278/1(d)
  bus_expand14/1(msb_out8) -> Gateway Out48/1
  Gateway Out122/1 -> To Workspace41/1
  Gateway Out123/1 -> To Workspace149/1
  Gateway Out124/1 -> To Workspace151/1
  bus_expand14/4(out5) -> Gateway Out124/1
  bus_expand14/3(out6) -> Gateway Out123/1
  bus_expand14/2(out7) -> Gateway Out122/1
  Gateway Out125/1 -> To Workspace152/1
  bus_expand14/5(out4) -> Gateway Out125/1
  Gateway Out126/1 -> To Workspace153/1
  bus_expand14/6(out3) -> Gateway Out126/1
  Gateway Out127/1 -> To Workspace154/1
  bus_expand14/7(out2) -> Gateway Out127/1
  Gateway Out128/1 -> To Workspace155/1
  bus_expand14/8(lsb_out1) -> Gateway Out128/1
  Slice34/1 -> bus_expand15/1(bus_in)
  [hmc_din_p0] -> pipeline279/1(d)
  Gateway Out129/1 -> To Workspace156/1
  Gateway Out130/1 -> To Workspace157/1
  Gateway Out131/1 -> To Workspace158/1
  Gateway Out132/1 -> To Workspace159/1
  Gateway Out133/1 -> To Workspace160/1
  Gateway Out134/1 -> To Workspace161/1
  Gateway Out135/1 -> To Workspace162/1
  Gateway Out136/1 -> To Workspace163/1
  bus_expand15/1(msb_out8) -> Gateway Out129/1
  bus_expand15/2(out7) -> Gateway Out130/1
  bus_expand15/3(out6) -> Gateway Out131/1
  bus_expand15/4(out5) -> Gateway Out132/1
  bus_expand15/5(out4) -> Gateway Out133/1
  bus_expand15/6(out3) -> Gateway Out134/1
  bus_expand15/7(out2) -> Gateway Out135/1
  bus_expand15/8(lsb_out1) -> Gateway Out136/1
  pipeline278/1(q) -> Slice35/1
  pipeline279/1(q) -> Slice34/1
  Gateway Out138/1 -> To Workspace166/1
  Gateway Out139/1 -> To Workspace167/1
  Gateway Out140/1 -> To Workspace168/1
  Gateway Out141/1 -> To Workspace169/1
  Delay81/1 -> delay10/1
  Constant1/1 -> [clear_hmc_addr_range]
  pipeline27/1(q) -> bus_expand5/1(bus_in)
  pipeline28/1(q) -> bus_expand8/1(bus_in)
  pipeline29/1(q) -> pipeline149/1(d)
  pipeline80/1(q) -> pipeline150/1(d), pipeline144/1(d)
  pipeline139/1(q) -> pipeline48/1(d)
  pipeline140/1(q) -> pipeline54/1(d), pipeline137/1(d)
  pipeline55/1(q) -> pipeline72/1(d)
  pipeline71/1(q) -> bus_expand2/1(bus_in)
  Gateway Out156/1 -> To Workspace183/1
  Gateway Out157/1 -> To Workspace184/1
  Gateway Out158/1 -> To Workspace185/1
  [hmc_reord_sync] -> delay4/1
  [hmc_reord_data] -> Slice38/1, Slice37/1
  Gateway Out160/1 -> To Workspace187/1
  Mux7/1 -> Gateway Out164/1, Slice36/1
  Gateway Out161/1 -> To Workspace188/1
  Gateway Out162/1 -> To Workspace189/1
  Gateway Out163/1 -> To Workspace190/1
  [hmc_reord_dvalid] -> delay3/1, [mux_sel], Gateway Out161/1, Mux7/1
  Slice36/1 -> Slice39/1, [fifo_dout], Gateway Out160/1
  Gateway Out164/1 -> To Workspace191/1
  Slice37/1 -> Gateway Out162/1, Mux7/2
  Slice38/1 -> Gateway Out163/1, Mux7/3
  Gateway Out165/1 -> To Workspace192/1
  bus_expand16/2(out7) -> Gateway Out167/1
  bus_expand16/3(out6) -> Gateway Out168/1
  bus_expand16/4(out5) -> Gateway Out169/1
  bus_expand16/5(out4) -> Gateway Out170/1
  bus_expand16/6(out3) -> Gateway Out171/1
  bus_expand16/7(out2) -> Gateway Out172/1
  bus_expand16/8(lsb_out1) -> Gateway Out173/1
  Gateway Out173/1 -> To Workspace200/1
  Gateway Out172/1 -> To Workspace199/1
  Gateway Out171/1 -> To Workspace198/1
  Gateway Out170/1 -> To Workspace197/1
  Gateway Out169/1 -> To Workspace196/1
  Gateway Out168/1 -> To Workspace194/1
  Gateway Out167/1 -> To Workspace203/1
  bus_expand16/1(msb_out8) -> Gateway Out174/1
  Gateway Out174/1 -> To Workspace195/1
  Slice39/1 -> bus_expand16/1(bus_in)
  Gateway Out206/1 -> To Workspace232/1
  Slice43/1 -> bus_expand19/1(bus_in)
  bus_expand19/1(msb_out8) -> Gateway Out206/1
  Gateway Out191/1 -> To Workspace233/1
  Gateway Out192/1 -> To Workspace218/1
  Gateway Out193/1 -> To Workspace219/1
  bus_expand19/4(out5) -> Gateway Out193/1
  bus_expand19/3(out6) -> Gateway Out192/1
  bus_expand19/2(out7) -> Gateway Out191/1
  Gateway Out194/1 -> To Workspace220/1
  bus_expand19/5(out4) -> Gateway Out194/1
  Gateway Out195/1 -> To Workspace221/1
  bus_expand19/6(out3) -> Gateway Out195/1
  Gateway Out196/1 -> To Workspace222/1
  bus_expand19/7(out2) -> Gateway Out196/1
  Gateway Out197/1 -> To Workspace223/1
  bus_expand19/8(lsb_out1) -> Gateway Out197/1
  Slice42/1 -> bus_expand20/1(bus_in)
  Gateway Out198/1 -> To Workspace224/1
  Gateway Out199/1 -> To Workspace225/1
  Gateway Out200/1 -> To Workspace226/1
  Gateway Out201/1 -> To Workspace227/1
  Gateway Out202/1 -> To Workspace228/1
  Gateway Out203/1 -> To Workspace229/1
  Gateway Out204/1 -> To Workspace230/1
  Gateway Out205/1 -> To Workspace231/1
  bus_expand20/1(msb_out8) -> Gateway Out198/1
  bus_expand20/2(out7) -> Gateway Out199/1
  bus_expand20/3(out6) -> Gateway Out200/1
  bus_expand20/4(out5) -> Gateway Out201/1
  bus_expand20/5(out4) -> Gateway Out202/1
  bus_expand20/6(out3) -> Gateway Out203/1
  bus_expand20/7(out2) -> Gateway Out204/1
  bus_expand20/8(lsb_out1) -> Gateway Out205/1
  Delay23/1 -> Delay10/1
  edge_detect29/1(out) -> Gateway Out165/1, [fifo_dvalid]
  delay3/1 -> edge_detect29/1(in)
  Gateway Out166/1 -> To Workspace193/1
  Gateway Out175/1 -> To Workspace201/1
  [ld_val] -> edge_detect30/1(in)
  Gateway Out176/1 -> To Workspace202/1
  edge_detect30/1(out) -> Register13/3, Gateway Out175/1
  [en_in] -> pipeline9/1(d), pipeline12/1(d)
  Gateway Out177/1 -> To Workspace204/1
  Gateway Out178/1 -> To Workspace205/1
  Gateway Out179/1 -> To Workspace206/1
  Logical10/1 -> Gateway Out179/1
  Gateway Out180/1 -> To Workspace207/1
  Delay9/1 -> [hmc_reord_dvalid], Gateway Out180/1
  Gateway Out181/1 -> To Workspace208/1
  [fifo_dvalid] -> pipeline15/1(d)
  pipeline15/1(q) -> pipeline57/1(d), pipeline269/1(d)
  [fifo_sync] -> pipeline37/1(d)
  pipeline37/1(q) -> pipeline270/1(d), pipeline56/1(d)
  Delay24/1 -> Delay81/1
  [hmc_rd_rdy] -> pipeline14/1(d)
  pipeline14/1(q) -> pipeline38/1(d)
  [hmc_wr_ready] -> pipeline39/1(d)
  pipeline39/1(q) -> pipeline40/1(d)
  pipeline40/1(q) -> hmc_debug1_p0/1(in_wr_rdy)
  pipeline96/1(q) -> hmc_debug1_p0/2(in_dvalid)
  pipeline38/1(q) -> hmc_debug1_p0/3(in_rd_rdy)
  pipeline100/1(q) -> hmc_debug1_p0/4(in_tag_out)
  pipeline42/1(q) -> hmc_debug1_p0/6(trig)
  pipeline41/1(q) -> hmc_debug1_p0/5(we)
  cd_hmc_sync_out_cnt1/1(sim_out) -> To Workspace2/1
  Counter8/1 -> pipeline44/1(d)
  pipeline44/1(q) -> cd_hmc_sync_out_cnt1/1(out_reg)
  pipeline45/1(q) -> Counter8/1
  pipeline43/1(q) -> Counter8/2
  edge_detect8/1 -> pipeline43/1(d)
  [hmc_waddr_p0] -> pipeline3/1(d)
  [hmc_raddr_p0] -> pipeline5/1(d)
  write_addr_gen_lnk3/1(addr_out) -> Gateway Out158/1, [hmc_clear_wraddr_pol1]
  Constant7/1 -> write_addr_gen_lnk3/2(offset)
  Constant17/1 -> write_addr_gen_lnk2/2(offset)
  write_addr_gen_lnk2/1(addr_out) -> Gateway Out157/1, [hmc_clear_wraddr_pol0]
  [hmc_post] -> Logical31/2
  [hmc_clear_done] -> Logical31/3
  [hmc_init] -> Logical31/1
  [hmc_wr_ready] -> Inverter1/1
  Inverter1/1 -> Logical2/1
  [hmc_win_p0] -> Logical2/2
  [hmc_rd_rdy] -> Inverter3/1
  Inverter3/1 -> Logical3/1
  [hmc_rin_p0] -> Logical3/2
  Logical2/1 -> Logical4/1
  Logical3/1 -> Logical4/2
  pipeline49/1(q) -> pipeline46/1(d)
  [hmc_tag_out] -> pipeline49/1(d)
  Logical4/1 -> [ss_stop]
  [ss_stop] -> hmc_debug1_p0/7(stop)
  edge_detect9/1(out) -> Convert2/1
  pipeline205/1(q) -> hmc_debug0_p0/1(in_win)
  pipeline201/1(q) -> hmc_debug0_p0/2(in_wr_rdy)
  pipeline204/1(q) -> hmc_debug0_p0/3(in_waddr)
  pipeline6/1(q) -> hmc_debug0_p0/4(in_rin)
  pipeline7/1(q) -> hmc_debug0_p0/5(in_rdaddr)
  pipeline8/1(q) -> hmc_debug0_p0/6(in_tag_in)
  pipeline46/1(q) -> hmc_debug0_p0/7(in_tag_out)
  pipeline99/1(q) -> hmc_debug0_p0/8(in_rd_rdy)
  pipeline178/1(q) -> hmc_debug0_p0/9(we)
  pipeline157/1(q) -> hmc_debug0_p0/10(trig)
  Constant6/1 -> hmc_din0_p0/11(stop), hmc_debug0_p0/11(stop), hmc_din1_p0/11(stop)
  Gateway Out10/1 -> To Workspace3/1
  Gateway Out12/1 -> To Workspace14/1
  pipeline50/1(q) -> Logical27/2
  [sys_rst] -> Gateway Out57/1, addr_stall/1, addr/1
  Gateway Out8/1 -> To Workspace15/1
  Gateway Out9/1 -> To Workspace34/1
  Gateway Out14/1 -> To Workspace35/1
  Delay10/1 -> second/3
  [sys_rst] -> second/2
  [ss_stop] -> Terminator/1
  edge_detect11/1 -> [sync_mon_rst]
  edge_detect24/1 -> pipeline175/1(d)
  edge_detect28/1 -> pipeline184/1(d)
  edge_detect33/1 -> pipeline166/1(d)
  [sys_rst] -> Register13/2
  [sys_rst] -> hmc_control/8(rst)
  [hmc_clear_done] -> Mux8/1
  [reord_clear_wraddr_pol0] -> Mux8/2
  [hmc_tag_out] -> Mux8/3
  Mux8/1 -> [reord_addr]
  [reord_addr] -> Gateway Out18/1, HMC_reord_bram/1
  [hmc_clear_done] -> Mux9/1
  [hmc_dout] -> Mux9/3
  Constant11/1 -> Mux9/2
  Mux9/1 -> [reord_data_in]
  [reord_data_in] -> Slice33/1, Slice32/1, Gateway Out11/1, HMC_reord_bram/2
  Mux10/1 -> [reord_wea]
  [hmc_dvalid] -> Mux10/3
  Constant19/1 -> Mux10/2
  [hmc_clear_done] -> Mux10/1
  Gateway Out5/1 -> To Workspace30/1
  Gateway Out15/1 -> To Workspace37/1
  Logical8/1 -> [hmc_clear_done]
  Register/1 -> Gateway Out41/1, Logical8/1
  reord_clear/1 -> Relational1/1, Gateway Out15/1, [reord_clear_wraddr_pol0]
  Constant21/1 -> Relational1/2
  Relational1/1 -> Register2/3, Register2/1
  Gateway Out17/1 -> To Workspace43/1
  Register2/1 -> Gateway Out17/1, Logical8/2
  Gateway Out18/1 -> To Workspace50/1
  Logical9/1 -> Gateway Out34/1, Reorder_cntrl/3(dvalid)
  [reord_wea] -> Logical9/1
  [hmc_clear_done] -> Delay7/1
  Gateway Out34/1 -> To Workspace51/1
  Delay7/1 -> Logical9/2
  Gateway Out41/1 -> To Workspace54/1
  Gateway Out16/1 -> To Workspace38/1
  Slice3/1 -> pipeline71/1(d)
  [hmc_clear_done] -> Mux11/1
  Mux11/1 -> Gateway Out44/1, [hmc_raddr_p0]
  Constant23/1 -> Mux11/2
  [hmc_raddr_pol0] -> Mux11/3
  Mux12/1 -> Gateway Out45/1, [hmc_tag_p0]
  [hmc_tag_pol0] -> Mux12/3
  Constant24/1 -> Mux12/2
  [hmc_clear_done] -> Mux12/1
  Mux13/1 -> Gateway Out50/1, [hmc_rin_p0]
  [hmc_rin_pol0] -> Mux13/3
  Constant25/1 -> Mux13/2
  [hmc_clear_done] -> Mux13/1
  [hmc_clear_done] -> Mux14/1
  Constant28/1 -> Mux14/2
  [hmc_raddr_pol1] -> Mux14/3
  [hmc_tag_pol1] -> Mux15/3
  Constant29/1 -> Mux15/2
  [hmc_clear_done] -> Mux15/1
  [hmc_rin_pol1] -> Mux16/3
  Constant30/1 -> Mux16/2
  [hmc_clear_done] -> Mux16/1
  Mux14/1 -> Gateway Out36/1, [hmc_raddr_p1]
  Mux15/1 -> Gateway Out40/1, [hmc_tag_p1]
  Mux16/1 -> Gateway Out43/1, [hmc_rin_p1]
  Gateway Out36/1 -> To Workspace52/1
  Gateway Out40/1 -> To Workspace53/1
  Gateway Out43/1 -> To Workspace55/1
  Gateway Out44/1 -> To Workspace56/1
  Gateway Out45/1 -> To Workspace57/1
  Gateway Out50/1 -> To Workspace58/1
  [hmc_rin_p0] -> pipeline62/1(d)
  [hmc_tag_pol0] -> pipeline59/1(d)
  [hmc_raddr_p0] -> pipeline60/1(d)
  [hmc_rd_rdy] -> pipeline58/1(d)
  pipeline58/1(q) -> pipeline190/1(d)
  pipeline59/1(q) -> pipeline189/1(d)
  pipeline60/1(q) -> pipeline188/1(d)
  pipeline62/1(q) -> pipeline187/1(d)
  [hmc_wr_ready] -> pipeline63/1(d)
  pipeline63/1(q) -> pipeline64/1(d)
  [hmc_win_p0] -> pipeline66/1(d)
  [hmc_waddr_p0] -> pipeline65/1(d)
  pipeline65/1(q) -> pipeline67/1(d)
  pipeline66/1(q) -> pipeline68/1(d)
  edge_detect7/1(out) -> pipeline51/1(d), pipeline47/1(d), pipeline13/1(d)
  Logical12/1 -> pipeline53/1(d), pipeline151/1(d), pipeline158/1(d), edge_detect7/1(in)
  bus_expand1/1(msb_out8) -> pipeline135/1(d)  "hmc_out1"
  bus_expand1/8(lsb_out1) -> pipeline148/1(d)  "hmc_out8"
  Slice11/1 -> bus_expand1/1(bus_in)
  bus_expand11/1(msb_out8) -> pipeline70/1(d)  "hmc_out9"
  bus_expand11/8(lsb_out1) -> pipeline134/1(d)  "hmc_out16"
  Slice17/1 -> bus_expand11/1(bus_in)
  pipeline135/1(q) -> hmc_din0_i/1(in_d00)
  pipeline136/1(q) -> hmc_din0_i/2(in_d01)
  pipeline141/1(q) -> hmc_din0_i/3(in_d02)
  pipeline143/1(q) -> hmc_din0_i/5(in_d04)
  pipeline145/1(q) -> hmc_din0_i/6(in_d05)
  pipeline147/1(q) -> hmc_din0_i/7(in_d06)
  pipeline151/1(q) -> hmc_din0_i/9(we)
  pipeline47/1(q) -> hmc_din0_i/10(trig)
  pipeline134/1(q) -> hmc_din1_i/8(in_d07)
  pipeline133/1(q) -> hmc_din1_i/7(in_d06)
  pipeline130/1(q) -> hmc_din1_i/6(in_d05)
  pipeline101/1(q) -> hmc_din1_i/5(in_d04)
  pipeline97/1(q) -> hmc_din1_i/4(in_d03)
  pipeline74/1(q) -> hmc_din1_i/3(in_d02)
  pipeline73/1(q) -> hmc_din1_i/2(in_d01)
  pipeline70/1(q) -> hmc_din1_i/1(in_d00)
  bus_expand1/2(out7) -> pipeline136/1(d)
  bus_expand1/4(out5) -> pipeline142/1(d)
  bus_expand1/7(out2) -> pipeline147/1(d)
  bus_expand1/3(out6) -> pipeline141/1(d)
  bus_expand11/7(out2) -> pipeline133/1(d)
  bus_expand1/5(out4) -> pipeline143/1(d)
  bus_expand1/6(out3) -> pipeline145/1(d)
  bus_expand11/5(out4) -> pipeline101/1(d)
  bus_expand11/4(out5) -> pipeline97/1(d)
  bus_expand11/6(out3) -> pipeline130/1(d)
  bus_expand11/3(out6) -> pipeline74/1(d)
  bus_expand11/2(out7) -> pipeline73/1(d)
  [hmc_din_p0] -> pipeline52/1(d), pipeline69/1(d)
  pipeline52/1(q) -> Slice17/1
  pipeline148/1(q) -> hmc_din0_i/8(in_d07)
  pipeline142/1(q) -> hmc_din0_i/4(in_d03)
  pipeline158/1(q) -> hmc_din1_i/9(we)
  pipeline51/1(q) -> hmc_din1_i/10(trig)
  pipeline69/1(q) -> Slice11/1
  pipeline179/1(q) -> pipeline163/1(d)
  [hmc_tag_p0] -> pipeline179/1(d)
  pipeline68/1(q) -> hmc_debug1/2(in_win)
  pipeline64/1(q) -> hmc_debug1/3(in_wr_rdy)
  pipeline187/1(q) -> hmc_debug1/6(in_rin)
  pipeline188/1(q) -> hmc_debug1/7(in_rdaddr)
  pipeline189/1(q) -> hmc_debug1/8(in_tag_in)
  pipeline163/1(q) -> hmc_debug1/9(in_tag_out)
  pipeline190/1(q) -> hmc_debug1/10(in_rd_rdy)
  pipeline53/1(q) -> hmc_debug1/13(we)
  pipeline13/1(q) -> hmc_debug1/14(trig)
  [hmc_init] -> Logical12/1
  [hmc_post] -> Logical12/2
  [hmc_clear_done] -> hmc_debug1/15(stop), hmc_din1_i/11(stop), hmc_din0_i/11(stop)
  pipeline191/1(q) -> hmc_debug1/1(in_clear_done)
  pipeline192/1(q) -> pipeline191/1(d)
  [hmc_clear_done] -> pipeline192/1(d)
  pipeline67/1(q) -> hmc_debug1/4(in_waddr_p0)
  pipeline218/1(q) -> hmc_debug1/5(in_waddr_p1)
  pipeline272/1(q) -> pipeline218/1(d)
  [hmc_waddr_p1] -> pipeline272/1(d)
  pipeline273/1(q) -> hmc_debug1/11(in_reord_addr)
  pipeline274/1(q) -> hmc_debug1/12(in_reord_wea)
  pipeline275/1(q) -> pipeline273/1(d)
  pipeline276/1(q) -> pipeline274/1(d)
  [reord_addr] -> pipeline275/1(d)
  [reord_wea] -> pipeline276/1(d)
  cd_hmc_clear_done/1(sim_out) -> To Workspace59/1
  [hmc_clear_done] -> cd_hmc_clear_done/1(out_reg)
  cd_hmc_clear_addr_cnt/1(sim_out) -> To Workspace60/1
  Counter1/1 -> cd_hmc_clear_addr_cnt/1(out_reg)
  pipeline282/1(q) -> Counter1/1
  pipeline281/1(q) -> Counter1/2
  [sys_rst] -> edge_detect34/1
  [hmc_clear_win] -> edge_detect10/1
  edge_detect34/1 -> pipeline282/1(d)
  edge_detect10/1 -> pipeline281/1(d)
  cd_hmc_clear_tp1/1(sim_out) -> To Workspace61/1
  Constant26/1 -> Relational2/2
  Register3/1 -> cd_hmc_clear_tp1/1(out_reg)
  Relational2/1 -> Register3/3, Register3/1
  cd_hmc_clear_tp2/1(sim_out) -> To Workspace62/1
  Register6/1 -> cd_hmc_clear_tp2/1(out_reg)
  Relational3/1 -> Register6/3, Register6/1
  Constant31/1 -> Relational3/2
  addr1/1 -> write_addr_gen_lnk3/1(addr_in), write_addr_gen_lnk2/1(addr_in), Gateway Out156/1, Relational2/1, Relational3/1, Relational/1
  cd_hmc_clear_tp3/1(sim_out) -> To Workspace63/1
  Register7/1 -> cd_hmc_clear_tp3/1(out_reg)
  Relational4/1 -> Register7/1, Register7/3
  Constant27/1 -> Relational4/2
  [hmc_clear_wraddr_pol1] -> Relational4/1
  edge_detect22/1 -> Register8/2, Register7/2, Register6/2, Register3/2, addr_stall1/1, Register/2, Register2/2, reord_clear/1, addr1/1, Gateway Out116/1
  cd_hmc_clear_tp4/1(sim_out) -> To Workspace64/1
  Register8/1 -> cd_hmc_clear_tp4/1(out_reg)
  Relational6/1 -> Register8/3, Register8/1
  Constant32/1 -> Relational6/2
  [hmc_clear_wraddr_pol0] -> Relational6/1
  [hmc_clear_done] -> Inverter4/1
  Inverter4/1 -> Logical7/3
  hmc/16 -> pipeline277/1(d)
  hmc/15 -> pipeline280/1(d)
  hmc/14 -> pipeline283/1(d)
  hmc/13 -> pipeline284/1(d)
  pipeline284/1(q) -> [rx_crc_err_lnk2]
  pipeline283/1(q) -> [rx_crc_err_lnk3]
  pipeline280/1(q) -> [errstat_lnk2]
  pipeline277/1(q) -> [errstat_lnk3]
  rx_crc_err_lnk2/1(sim_out) -> To Workspace65/1
  [rx_crc_err_lnk2] -> rx_crc_err_lnk2/1(out_reg)
  rx_crc_err_lnk3/1(sim_out) -> To Workspace66/1
  [rx_crc_err_lnk3] -> rx_crc_err_lnk3/1(out_reg)
  [errstat_lnk3] -> errstat_lnk3/1(out_reg)
  [errstat_lnk2] -> errstat_lnk2/1(out_reg)
  errstat_lnk2/1(sim_out) -> To Workspace78/1
  errstat_lnk3/1(sim_out) -> To Workspace79/1
  [hmc_clear_done] -> Logical13/2
  Logical13/1 -> Terminator1/1
  Gateway Out57/1 -> To Workspace80/1
